simulink model "speedDistRegulator"  (R2017b)
settings: configuration reference "ControlDesignConfigSet" (kept outside this file)
libraries: simulink x1
settings Model: Creator=eh6qym  LastModifiedBy=dkw1dx
settings ConfigSetRef: SourceLocation=Base Workspace

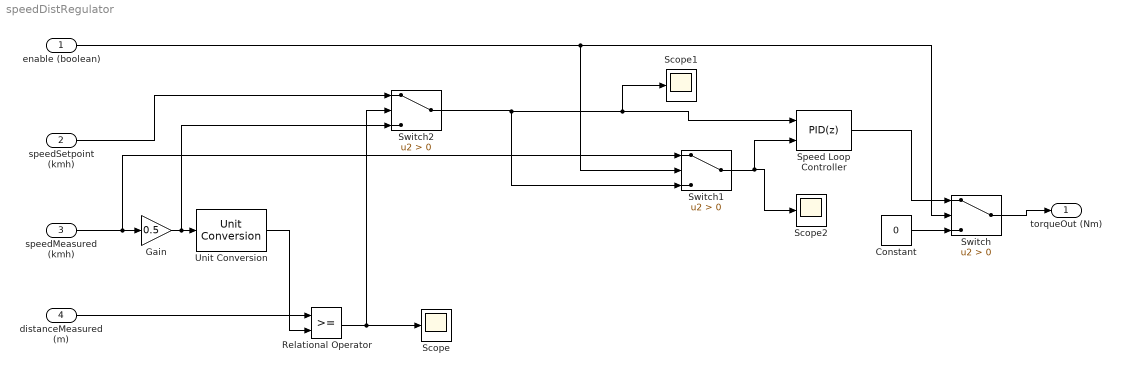
== system speedDistRegulator ==
  enable (boolean) : Inport  OutDataTypeStr=boolean
  speedSetpoint (kmh) : Inport  Port=2  OutDataTypeStr=double  Unit=kmh
  speedMeasured (kmh) : Inport  Port=3  OutDataTypeStr=double  Unit=kmh
  distanceMeasured (m) : Inport  Port=4  OutDataTypeStr=double  Unit=kmh
  Constant : Constant  Value=0
  Gain : Gain  Gain=0.5
  Relational Operator : RelationalOperator  OutDataTypeStr=boolean  RndMeth=Simplest  InputSameDT=on
  Scope : Scope
  Scope1 : Scope
  Scope2 : Scope
  Speed Loop Controller : simulink/Continuous/PID Controller (2DOF)  Controller=PID  TimeDomain=Discrete-time  SampleTime=-1  IntegratorMethod=Forward Euler  FilterMethod=Forward Euler  Form=Parallel  UseFilter=on  ControllerParametersSource=internal  P=0.117306022501173  I=1.17306022501173  D=0  N=100  b=1  c=1  InitialConditionSource=internal  InitialConditionForIntegrator=0  InitialConditionForFilter=0  ExternalReset=none  LimitOutput=on  UpperSaturationLimit=200  LowerSaturationLimit=0  LinearizeAsGain=on  AntiWindupMode=clamping  Kb=1  TrackingMode=off  Kt=1  PParamMin=[]  PParamMax=[]  IParamMin=[]  IParamMax=[]  DParamMin=[]  DParamMax=[]  NParamMin=[]  NParamMax=[]  bParamMin=[]  bParamMax=[]  cParamMin=[]  cParamMax=[]  KbParamMin=[]  KbParamMax=[]  KtParamMin=[]  KtParamMax=[]  POutMin=[]  POutMax=[]  IOutMin=[]  IOutMax=[]  DOutMin=[]  DOutMax=[]  NOutMin=[]  NOutMax=[]  bOutMin=[]  bOutMax=[]  cOutMin=[]  cOutMax=[]  KbOutMin=[]  KbOutMax=[]  KtOutMin=[]  KtOutMax=[]  IntegratorOutMin=[]  IntegratorOutMax=[]  FilterOutMin=[]  FilterOutMax=[]  SumOutMin=[]  SumOutMax=[]  Sum1OutMin=[]  Sum1OutMax=[]  Sum2OutMin=[]  Sum2OutMax=[]  Sum3OutMin=[]  Sum3OutMax=[]  SumI1OutMin=[]  SumI1OutMax=[]  SumI2OutMin=[]  SumI2OutMax=[]  SumI3OutMin=[]  SumI3OutMax=[]  SumDOutMin=[]  SumDOutMax=[]  SaturationOutMin=[]  SaturationOutMax=[]  IntegratorContinuousStateAttributes=''  IntegratorStateMustResolveToSignalObject=off  IntegratorRTWStateStorageClass=Auto  FilterContinuousStateAttributes=''  FilterStateMustResolveToSignalObject=off  FilterRTWStateStorageClass=Auto  DifferentiatorICPrevScaledInput=0  DifferentiatorOutMin=[]  DifferentiatorOutMax=[]  InitialConditionSetting=State (most efficient)  FilterDiffOutCoefMin=[]  FilterDiffOutCoefMax=[]  SumDenOutMin=[]  SumDenOutMax=[]  SumNumOutMin=[]  SumNumOutMax=[]  ReciprocalOutMin=[]  ReciprocalOutMax=[]  DivideOutMin=[]  DivideOutMax=[]  TunerSelectOption=Transfer Function Based (PID Tuner App)
  Switch : Switch  Criteria=u2 > Threshold
  Switch1 : Switch  Criteria=u2 > Threshold
  Switch2 : Switch  Criteria=u2 > Threshold
  Unit Conversion : UnitConversion
  torqueOut (Nm) : Outport  OutDataTypeStr=double  Unit=Nm
  wires:
  speedMeasured (kmh)/1 -> Switch1/1, Gain/1
  Gain/1 -> Switch2/3, Unit Conversion/1
  Constant/1 -> Switch/3
  Switch/1 -> torqueOut (Nm)/1
  Speed Loop Controller/1 -> Switch/1
  enable (boolean)/1 -> Switch1/2, Switch/2
  Switch1/1 -> Scope2/1, Speed Loop Controller/2
  distanceMeasured (m)/1 -> Relational Operator/1
  Unit Conversion/1 -> Relational Operator/2
  Switch2/1 -> Scope1/1, Speed Loop Controller/1, Switch1/3
  speedSetpoint (kmh)/1 -> Switch2/1
  Relational Operator/1 -> Scope/1, Switch2/2
